simulink model "exercise2_2SIM"  (R2025b)
settings: Solver=VariableStepAuto  StartTime=0.0  StopTime=100  RelTol=1e-3
values from neighbouring files (symbols this model uses):
  A = [   0,                                        1,            0,                                              0,    0 ... (first row only)    [Exercise1.m]    (also in Exercise_2.m = [   0,  1,           0,  0,    0; symbolic_state_space_gen.m = jacobian(dx, x))
  B = [                           0 ... (first row only)    [Exercise1.m]    (also in Exercise_2.m = [0,     0; symbolic_state_space_gen.m = jacobian(dx, u))
  c = 1500    [Exercise1.m]    (also in Exercise_2.m; exercise_3.m)
  C = [-K/ms, -(2*zeta0*(K*ms)^(1/2) + 2*zeta_d*(K*ms)^(1/2))/ms, K/ms, (2*zeta0*(K*ms)^(1/2) - 2*zeta_d*(K*ms)^(1/2))/ms, 0 ... (first row only)    [Exercise1.m]    (also in Exercise_2.m = [-K/ms, 0, K/ms, 0, 0; symbolic_state_space_gen.m = jacobian(y, x))
  c_max = 4000    [Exercise_2.m]
  cs = cs_tune(i)    [Exercise_2.m]
  D = [                        0 ... (first row only)    [Exercise1.m]    (also in Exercise_2.m = [0, 1/ms; symbolic_state_space_gen.m = jacobian(y, u))
  V = 20    [Exercise_2.m]
libraries: simulink x1
settings Model: Creator=carlonovara  LastModifiedBy=denni
settings SolverCC: AlgebraicLoopSolver=TrustRegion
settings DataIOCC: ReturnWorkspaceOutputs=off
settings DebuggingCC: UnconnectedInputMsg=warning  UnconnectedOutputMsg=warning  UnconnectedLineMsg=warning
settings ModelReferenceCC: EnableRefExpFcnMdlSchedulingChecks=on
settings RTWCC: GPUComputeCapability=3.5  DLArmComputeVersion=19.05

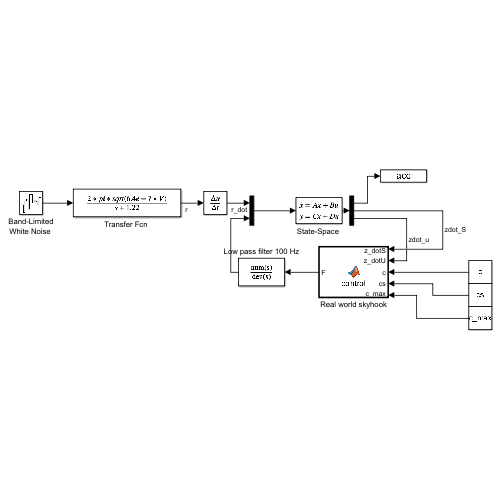
[thumbnail: Simulink's stored preview of the top-level diagram]
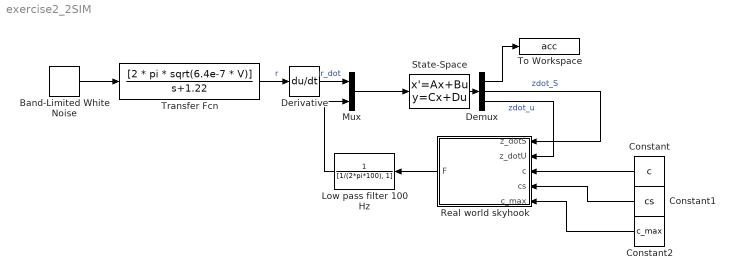
== system exercise2_2SIM ==
  "Band-Limited White Noise " : simulink/Sources/Band-Limited White Noise  Cov=1  Ts=0.05  seed=0019234
  Constant : Constant  Value=c
  Constant1 : Constant  Value=cs
  Constant2 : Constant  Value=c_max
  Demux : Demux  Outputs=3
  Derivative : Derivative
  Low pass filter 100 Hz : TransferFcn  Denominator=[1/(2*pi*100), 1]
  Mux : Mux  Inputs=2
  Real world skyhook : MATLAB Function  TreatAsAtomicUnit=on
  "State-Space " : StateSpace  A=A  B=B  C=C  D=D  InitialCondition=0
  To Workspace : ToWorkspace  VariableName=acc  SampleTime=-1
  "Transfer Fcn " : TransferFcn  Numerator=[2 * pi * sqrt(6.4e-7 * V)]  Denominator=[1 1.22]
  wires:
  "State-Space "/1 -> Demux/1
  Demux/2 -> Real world skyhook/1(z_dotS)  "zdot_S"
  Demux/3 -> Real world skyhook/2(z_dotU)  "zdot_u"
  Mux/1 -> "State-Space "/1
  Demux/1 -> To Workspace/1
  Constant/1 -> Real world skyhook/3(c)
  Constant1/1 -> Real world skyhook/4(cs)
  Constant2/1 -> Real world skyhook/5(c_max)
  Real world skyhook/1(F) -> Low pass filter 100 Hz/1
  Low pass filter 100 Hz/1 -> Mux/2
  "Band-Limited White Noise "/1 -> "Transfer Fcn "/1
  Derivative/1 -> Mux/1  "r_dot"
  "Transfer Fcn "/1 -> Derivative/1  "r"

== matlab function exercise2_2SIM/Real world skyhook ==
  data: z_dotS input; F output; z_dotU input; c input; cs input; c_max input
function F = control(z_dotS, z_dotU, c, cs, c_max)
    if z_dotS * (z_dotS-z_dotU)>0
        F_req = -(cs+c) * z_dotS + c* z_dotU;
    else F_req = -c * (z_dotS-z_dotU);
    end

    % constraint application   c *v_rel < F < c_max * v_rel
    v_rel = z_dotS-z_dotU;
    F_min = -c*v_rel;
    F_max = -c_max*v_rel;
    if v_rel < 0
        F = min (F_max, max(F_req, F_min) );
    elseif v_rel >0
        F = max ( F_min, min ( F_req, F_max) );
    else 
        F = 0;

    end
end
